simulink model "Channel"  (R2023b)
settings: Solver=VariableStepAuto  StartTime=0.0  StopTime=0.01  MaxStep=1e-3  RelTol=1e-3
libraries: simulink x6, dspsrcs4 x1, dspsigops x1
(part 1 of 3)
settings Model: Creator=Sepiamw  LastModifiedBy=Armin
settings DebuggingCC: UnconnectedInputMsg=warning  UnconnectedOutputMsg=warning  UnconnectedLineMsg=warning
settings ModelReferenceCC: EnableRefExpFcnMdlSchedulingChecks=on
settings RTWCC: DLArmComputeVersion=19.05

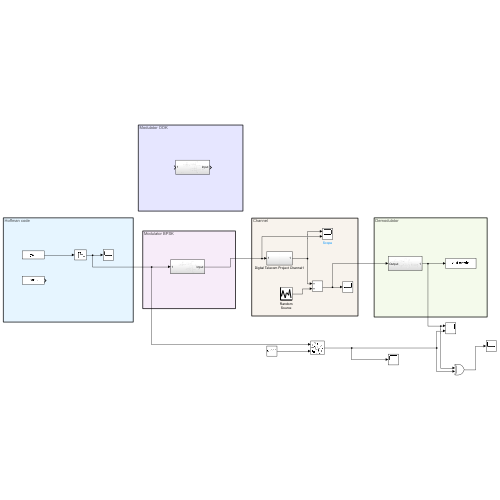
[thumbnail: Simulink's stored preview of the top-level diagram]
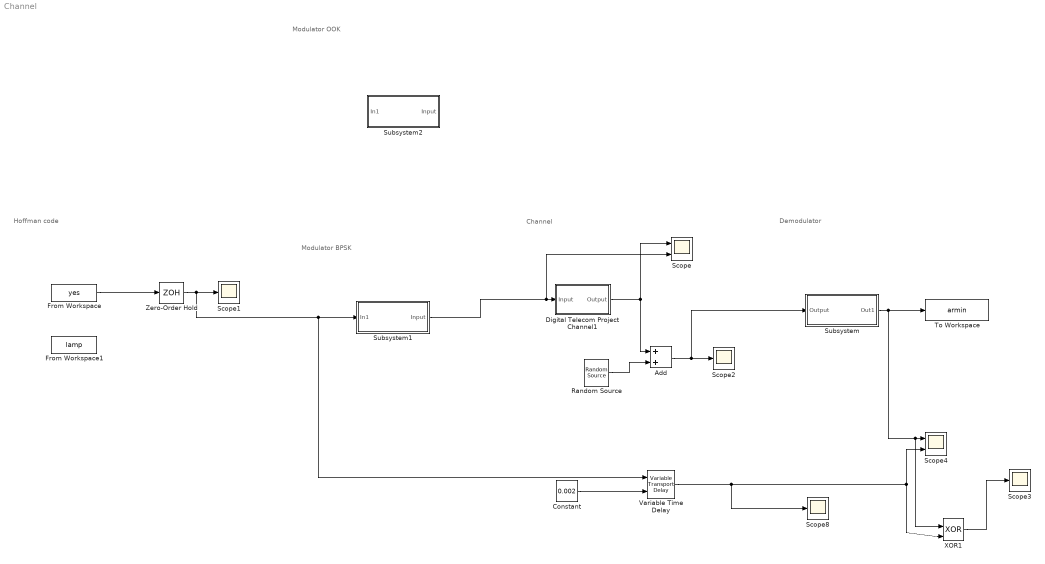
== system Channel ==
  note: Modulator OOK
  note: Demodulator
  note: Channel
  note: Modulator BPSK
  note: Hoffman code
  Add : Sum
  Constant : Constant  Value=0.002
  Digital Telecom Project Channel1 : Subsystem  Tag=FilterWizardSubSystem
      settings: ErrorFcn=dspFilterRealizedInBasicElemsAlgLoopErrFcnCallback
  From Workspace : FromWorkspace  VariableName=yes  OutDataTypeStr=double  SampleTime=1e-3
  From Workspace1 : FromWorkspace  VariableName=lamp  OutDataTypeStr=double  SampleTime=1e-3
  Random Source : dspsrcs4/Random Source  SrcType=Gaussian  NormMethod=Ziggurat  CltLength=12  MinVal=0  MaxVal=1  MeanVal=0  VarVal=2000  RepMode=Not repeatable  rawSeed=1  IsInherit=off  SampMode=Discrete  SampTime=1e-5  SampFrame=1  DataType=Double  OutComplex=Real  OutputFrames=off
  Scope : Scope  NumInputPorts=2
  Scope{1..3,8} (4 alike) : Scope
  Scope4 : Scope  NumInputPorts=2
  Subsystem : Subsystem
  Subsystem1 : Subsystem
  Subsystem2 : Subsystem
  To Workspace : ToWorkspace  VariableName=armin  SampleTime=1e-5
      settings: Save2DSignal=2-D array (concatenate along first dimension)
  Variable Time Delay : VariableTransportDelay  MaximumDelay=10
  XOR1 : Logic  Operator=XOR  IconShape=distinctive  AllPortsSameDT=off  OutDataTypeStr=boolean
  Zero-Order Hold : ZeroOrderHold  SampleTime=1e-3
  wires:
  Zero-Order Hold/1 -> Variable Time Delay/1, Subsystem1/1(In1), Scope1/1
  Subsystem1/1(Input) -> Scope/2, Digital Telecom Project Channel1/1(Input)
  Digital Telecom Project Channel1/1(Output) -> Add/1, Scope/1
  Random Source/1 -> Add/2
  Add/1 -> Scope2/1, Subsystem/1(Output)
  Variable Time Delay/1 -> Scope8/1, XOR1/2, Scope4/2
  Constant/1 -> Variable Time Delay/2
  Subsystem/1(Out1) -> XOR1/1, Scope4/1, To Workspace/1
  From Workspace/1 -> Zero-Order Hold/1
  XOR1/1 -> Scope3/1
